simulink model "vertical_smm_with_lqr_3d"  (R2014b)
settings: Solver=FixedStepDiscrete  StartTime=0.0  StopTime=inf  FixedStep=sample_time  RelTol=1e-3
values from neighbouring files (symbols this model uses):
  forward_dx = [-0.304875592207 -0.274388032987 -0.243900473766 -0.213412914545 -0.182925355324 -0.152437796104 -0.121950236883 -0.0914626776622 -0.0609751184415 -0.0304875592207 0 0.0304875592207 ... (714 elements, 21x34)]    [ref_trajs.mat]
  forward_dx_of_dxstar = [-1.3048755994 -1.25487559904 -1.20487559868 -1.15487559832 -1.10487559796 -1.0548755976 -1.00487559724 -0.954875596883 -0.904875596523 -0.854875596164 -0.804875595804 -0.754875595707 ... (29274 elements, 41x21x34)]    [ref_trajs.mat]
  forward_x = [0.0961104217981 0.0864993796183 0.0768883374385 0.0672772952586 0.0576662530788 0.048055210899 0.0384441687192 0.0288331265394 0.0192220843596 0.00961104217981 0 -0.00961104217981 ... (714 elements, 21x34)]    [ref_trajs.mat]
  forward_x_of_dxstar = [0.247353819189 0.239791649319 0.232229479449 0.22466730958 0.21710513971 0.209542969841 0.201980799971 0.194418630102 0.186856460232 0.179294290363 0.171732120493 0.164169950675 ... (29274 elements, 41x21x34)]    [ref_trajs.mat]
  target_dx_range = [-1 -0.95 -0.9 -0.85 -0.8 -0.75 -0.7 -0.65 -0.6 -0.55 -0.5 -0.45 ... (41 elements, 1x41)]    [ref_trajs.mat]
undefined symbols (not defined in the file or in its folder): A_kalman_fourbar_gear, A_kalman_transverse, A_kalman_vertical, A_lpf_dtau, A_lpf_leg_spring, B1_lpf_dtau, B1_lpf_leg_spring, B2_lpf_dtau, B2_lpf_leg_spring, B_dx_versus_x0, B_kalman_fourbar_gear, B_kalman_transverse, B_kalman_vertical, backwards_K_front_of_t_row1, backwards_K_front_of_t_row2, backwards_K_sag_of_t, C_kalman_fourbar_gear, C_kalman_transverse, C_kalman_vertical, com_leg_motor, com_torso, contact_threshold, control_start_time, d_vertical_com, deadbeat_enabled, desired_com_forward_velocity, desired_com_lateral_velocity, desired_initial_leg_roll_left, desired_initial_leg_roll_right, desired_lateral_symmetry_angle, desired_torso_pitch, desired_torso_roll, Discrete, fcut_contact, forward_velocity_target_step, g, HIP_MTR_MAX_CONT_TORQUE, i_leg_motor, i_robot, i_torso, initial_dx_estimate, initial_dy_estimate, initial_dz_estimate, initial_z_estimate, j_motor, j_segments, K_left_lat_flight, K_left_lat_flight_winch, k_LQR_vertical, K_right_lat_flight, K_right_lat_flight_winch, k_sea, k_vertical_winch, kalman_load_to_deflect_transmission, kalman_stance_slip_threshold, kd_motor, kp_motor, l_retract_delta, l_retract_swing_max, l_retract_swing_min ... (+58)
libraries: simulink x8, ctrlSharedLib x7
(part 3 of 4)

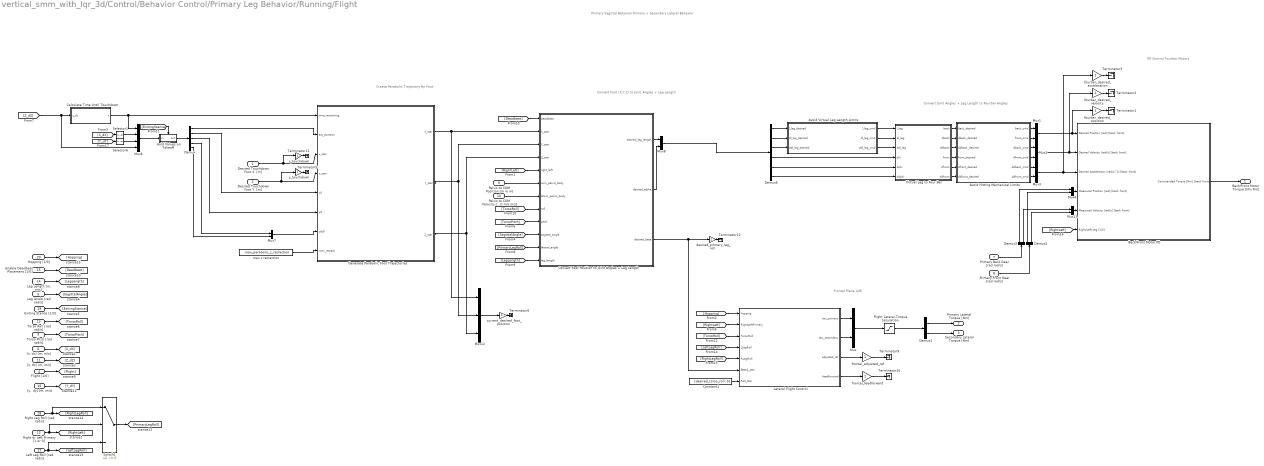
== system vertical_smm_with_lqr_3d/Control/Behavior Control/Primary Leg Behavior/Running/Flight ==
  note: Primary Sagittal Behavior
      | Primary + Secondary Lateral Behavior
  note: Create Parabolic
      | Trajectory for Foot
  note: Convert Foot (X,Y,Z) to
      | Joint Angles + Leg Length
  note: Convert Joint Angles + Leg Length
      | to Fourbar Angles
  note: PD Control Fourbar Motors
  note: Frontal Plane LQR
  Desired Touchdown Foot X  [m] : Inport
  Desired Touchdown Foot Y  [m] : Inport  Port=2
  Torso Pitch [rad rad/s] : Inport  Port=3
  Flight [1/0] : Inport  Port=4
  Leg Angle [rad rad/s] : Inport  Port=5
  "[x, dx] [m, m/s]" : Inport  Port=6
  Primary Back Gear [rad rad/s] : Inport  Port=7
  Primary Front Gear [rad rad/s] : Inport  Port=8
  Pelvis to COM Position [m m m] : Inport  Port=9
  Pelvis to COM Velocity [m/s m/s m/s] : Inport  Port=10
  "[z, dz] [m, m/s]" : Inport  Port=11
  Right or Left Primary [1 or 0] : Inport  Port=12
  Torso Roll [rad rad/s] : Inport  Port=13
  "Leg Length [m, m/s]" : Inport  Port=14
  Enable Deadbeat Placement [1/0] : Inport  Port=15
  "[y,  dy] [m, m/s]" : Inport  Port=16
  "Left Leg Roll [rad, rad/s]" : Inport  Port=17
  "Right Leg Roll [rad, rad/s]" : Inport  Port=18
  Exiting Stance [1/0] : Inport  Port=19
  Hopping [1/0] : Inport  Port=20
  Avoid Hitting Mechanical Limits : MATLAB Function  TreatAsAtomicUnit=on
  Avoid Virtual Leg Length Limits : MATLAB Function  TreatAsAtomicUnit=on
  Back/Front Motor PD : Subsystem
  Calculate Time Until Touchdown : MATLAB Function  TreatAsAtomicUnit=on
  Constant1 : Constant  Value=[desired_torso_roll; 0]
  "Convert Foot Position to Joint Angles + Leg Length " : MATLAB Function  TreatAsAtomicUnit=on
  Demux : Demux  Outputs=5
  Demux1 : Demux  Outputs=2
  Demux2 : Demux  Outputs=2
  Demux3 : Demux  Outputs=2
  Demux6 : Demux  Outputs=6
  Flight Lateral Torque Saturation : Saturate  UpperLimit=HIP_MTR_MAX_CONT_TORQUE  LowerLimit=-HIP_MTR_MAX_CONT_TORQUE
      settings: AttributesFormatString=Top: %<UpperLimit>\nBottom: %<LowerLimit>
  Generate Parabolic Foot Trajectories : MATLAB Function  TreatAsAtomicUnit=on
  Hold Values on Takeoff : Subsystem
  Lateral Flight Control : MATLAB Function  TreatAsAtomicUnit=on
  Mux{,1..4,7..8,11} (8 alike) : Mux  Inputs=2
  Mux12 : Mux  Inputs=3
  Mux6 : Mux
  Selector1 : Selector  InputPortWidth=2  Indices=[1]
  Selector6 : Selector  InputPortWidth=2  Indices=[1]
  Switch1 : Switch  Criteria=u2 ~= 0
  Terminator{1..3,5..6,9..12} (9 alike) : Terminator
  Virtual Leg to Four Bar : MATLAB Function  TreatAsAtomicUnit=on
  current_desired_foot_position : Gain
  desired_primary_leg_roll : Gain
  fourbar_desired_acceleration : Gain
  fourbar_desired_position : Gain
  fourbar_desired_velocity : Gain
  frontal_adjusted_ref : Gain
  frontal_feedforward : Gain
  max z retraction : Constant  Value=max_parabolic_z_retraction
  x_touchdown : Gain
  y_touchdown : Gain
  Back/Front Motor Torque [Nm Nm] : Outport
  Primary Lateral Torque [Nm] : Outport  Port=2
  Secondary Lateral Torque [Nm] : Outport  Port=3
  wires:
  Virtual Leg to Four Bar/1(back) -> Avoid Hitting Mechanical Limits/1(back_desired)
  Virtual Leg to Four Bar/2(dback) -> Avoid Hitting Mechanical Limits/2(dback_desired)
  Virtual Leg to Four Bar/3(ddback) -> Avoid Hitting Mechanical Limits/3(ddback_desired)
  Virtual Leg to Four Bar/4(front) -> Avoid Hitting Mechanical Limits/4(front_desired)
  Virtual Leg to Four Bar/5(dfront) -> Avoid Hitting Mechanical Limits/5(dfront_desired)
  Virtual Leg to Four Bar/6(ddfront) -> Avoid Hitting Mechanical Limits/6(ddfront_desired)
  Mux11/1 -> Back/Front Motor PD/5(Measured Velocity [rad/s] [back front])
  Demux2/2 -> Mux11/2
  Mux4/1 -> Back/Front Motor PD/4(Measured Position [rad] [back front])
  Mux1/1 -> fourbar_desired_position/1, Back/Front Motor PD/1(Desired Position [rad] [back front])
  Demux3/2 -> Mux11/1
  Demux3/1 -> Mux4/1
  Avoid Hitting Mechanical Limits/2(front_cmd) -> Mux1/2
  Avoid Hitting Mechanical Limits/1(back_cmd) -> Mux1/1
  Demux2/1 -> Mux4/2
  Avoid Hitting Mechanical Limits/3(dback_cmd) -> Mux2/1
  Avoid Hitting Mechanical Limits/4(dfront_cmd) -> Mux2/2
  Avoid Hitting Mechanical Limits/5(ddback_cmd) -> Mux3/1
  Avoid Hitting Mechanical Limits/6(ddfront_cmd) -> Mux3/2
  Mux2/1 -> fourbar_desired_velocity/1, Back/Front Motor PD/2(Desired Velocity [rad/s] [back front])
  Mux3/1 -> fourbar_desired_acceleration/1, Back/Front Motor PD/3(Desired Acceleration [rad/s^2] [back front])
  Back/Front Motor PD/1(Commanded Torque [Nm] [back front]) -> Back/Front Motor Torque [Nm Nm]/1
  Primary Back Gear [rad rad/s]/1 -> Demux3/1
  Primary Front Gear [rad rad/s]/1 -> Demux2/1
  [RightLeft] -> Back/Front Motor PD/6(Right/Left Leg [1/0])
  fourbar_desired_position/1 -> Terminator1/1
  fourbar_desired_velocity/1 -> Terminator2/1
  fourbar_desired_acceleration/1 -> Terminator3/1
  Demux/1 -> Generate Parabolic Foot Trajectories/2(est_duration)
  Mux7/1 -> Generate Parabolic Foot Trajectories/7(zdz0)
  max z retraction/1 -> Generate Parabolic Foot Trajectories/8(max_retract)
  Mux6/1 -> Hold Values on Takeoff/1(in)
  Hold Values on Takeoff/1(out) -> Demux/1
  Selector1/1 -> Mux6/2
  [X_dX] -> Selector1/1
  Generate Parabolic Foot Trajectories/1(X_star) -> Mux12/1, "Convert Foot Position to Joint Angles + Leg Length "/2(X_star)
  Generate Parabolic Foot Trajectories/2(Y_star) -> "Convert Foot Position to Joint Angles + Leg Length "/3(Y_star), Mux12/2
  Generate Parabolic Foot Trajectories/3(Z_star) -> "Convert Foot Position to Joint Angles + Leg Length "/4(Z_star), Mux12/3
  [RightLeft] -> "Convert Foot Position to Joint Angles + Leg Length "/5(right_left)
  "Convert Foot Position to Joint Angles + Leg Length "/2(desired_alpha) -> Mux8/2
  "Convert Foot Position to Joint Angles + Leg Length "/1(desired_leg_length) -> Mux8/1
  Demux6/6 -> Virtual Leg to Four Bar/6(ddphi)
  Demux6/5 -> Virtual Leg to Four Bar/5(dphi)
  Demux6/4 -> Virtual Leg to Four Bar/4(phi)
  Mux8/1 -> Demux6/1
  Leg Angle [rad rad/s]/1 -> [SagittalAngle]
  [SagittalAngle] -> "Convert Foot Position to Joint Angles + Leg Length "/10(sagittal_angle)
  Torso Pitch [rad rad/s]/1 -> [TorsoPitch]
  [TorsoPitch] -> "Convert Foot Position to Joint Angles + Leg Length "/9(pitch)
  [PrimaryLegRoll] -> "Convert Foot Position to Joint Angles + Leg Length "/11(lateral_angle)
  [LegLength] -> "Convert Foot Position to Joint Angles + Leg Length "/12(leg_length)
  [TorsoRoll] -> "Convert Foot Position to Joint Angles + Leg Length "/8(roll)
  Pelvis to COM Position [m m m]/1 -> "Convert Foot Position to Joint Angles + Leg Length "/6(com_pelvis_body)
  Pelvis to COM Velocity [m/s m/s m/s]/1 -> "Convert Foot Position to Joint Angles + Leg Length "/7(dcom_pelvis_body)
  Flight [1/0]/1 -> [Flight]
  [ExitingStance] -> Hold Values on Takeoff/Trigger
  "[x, dx] [m, m/s]"/1 -> [X_dX]
  Torso Roll [rad rad/s]/1 -> [TorsoRoll]
  "Leg Length [m, m/s]"/1 -> [LegLength]
  Enable Deadbeat Placement [1/0]/1 -> [Deadbeat]
  "[z, dz] [m, m/s]"/1 -> [Z_dZ]
  Desired Touchdown Foot X  [m]/1 -> x_touchdown/1, Generate Parabolic Foot Trajectories/3(x_star)
  x_touchdown/1 -> Terminator11/1
  y_touchdown/1 -> Terminator5/1
  current_desired_foot_position/1 -> Terminator6/1
  Mux12/1 -> current_desired_foot_position/1
  "[y,  dy] [m, m/s]"/1 -> [Y_dY]
  [Y_dY] -> Selector6/1
  [Z_dZ] -> Mux6/4, Calculate Time Until Touchdown/1(z_dz)
  Selector6/1 -> Mux6/3
  Demux/2 -> Generate Parabolic Foot Trajectories/5(x0)
  Demux/3 -> Generate Parabolic Foot Trajectories/6(y0)
  Demux/4 -> Mux7/1
  Demux/5 -> Mux7/2
  Calculate Time Until Touchdown/1(t) -> Mux6/1, Generate Parabolic Foot Trajectories/1(time_remaining)
  Avoid Virtual Leg Length Limits/1(l_leg_cmd) -> Virtual Leg to Four Bar/1(l_leg)
  Avoid Virtual Leg Length Limits/2(dl_leg_cmd) -> Virtual Leg to Four Bar/2(dl_leg)
  Avoid Virtual Leg Length Limits/3(ddl_leg_cmd) -> Virtual Leg to Four Bar/3(ddl_leg)
  Demux6/1 -> Avoid Virtual Leg Length Limits/1(l_leg_desired)
  Demux6/2 -> Avoid Virtual Leg Length Limits/2(dl_leg_desired)
  Demux6/3 -> Avoid Virtual Leg Length Limits/3(ddl_leg_desired)
  Desired Touchdown Foot Y  [m]/1 -> y_touchdown/1, Generate Parabolic Foot Trajectories/4(y_star)
  [RightLeft] -> Lateral Flight Control/2(RightLeftPrimary)
  [TorsoRoll] -> Lateral Flight Control/3(TorsoRoll)
  Constant1/1 -> Lateral Flight Control/7(Roll_star)
  Lateral Flight Control/3(adjusted_ref) -> frontal_adjusted_ref/1
  Lateral Flight Control/4(feedforward) -> frontal_feedforward/1
  Lateral Flight Control/2(tau_secondary) -> Mux/2
  Lateral Flight Control/1(tau_primary) -> Mux/1
  "Left Leg Roll [rad, rad/s]"/1 -> Switch1/3, [LeftLegRoll]
  [LeftLegRoll] -> Lateral Flight Control/4(LLegRoll)
  [RightLegRoll] -> Lateral Flight Control/5(RLegRoll)
  "Right Leg Roll [rad, rad/s]"/1 -> Switch1/1, [RightLegRoll]
  Right or Left Primary [1 or 0]/1 -> Switch1/2, [RightLeft]
  Switch1/1 -> [PrimaryLegRoll]
  Exiting Stance [1/0]/1 -> [ExitingStance]
  Demux1/1 -> Primary Lateral Torque [Nm]/1
  Demux1/2 -> Secondary Lateral Torque [Nm]/1
  desired_primary_leg_roll/1 -> Terminator12/1
  "Convert Foot Position to Joint Angles + Leg Length "/3(desired_beta) -> Lateral Flight Control/6(Beta1_star), desired_primary_leg_roll/1
  Flight Lateral Torque Saturation/1 -> Demux1/1
  frontal_feedforward/1 -> Terminator10/1
  frontal_adjusted_ref/1 -> Terminator9/1
  [Deadbeat] -> "Convert Foot Position to Joint Angles + Leg Length "/1(deadbeat)
  Mux/1 -> Flight Lateral Torque Saturation/1
  [Hopping] -> Lateral Flight Control/1(hopping)
  Hopping [1/0]/1 -> [Hopping]

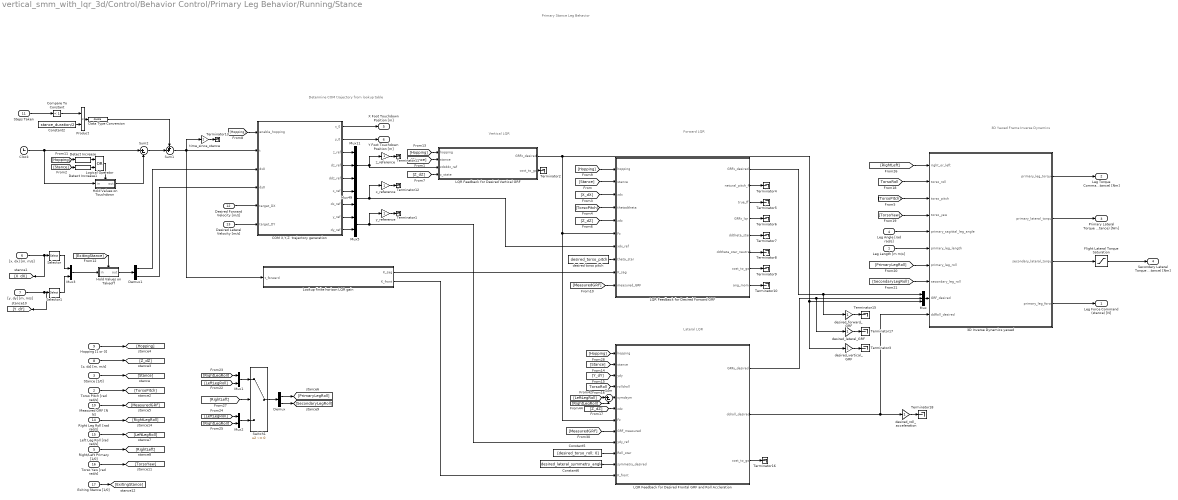
== system vertical_smm_with_lqr_3d/Control/Behavior Control/Primary Leg Behavior/Running/Stance ==
  note: Primary Stance Leg Behavior
  note: Determine COM trajectory
      | from lookup table
  note: Vertical LQR
  note: Forward LQR
  note: 3D Yawed Frame Inverse Dynamics
  note: Lateral LQR
  Leg Length [m m/s] : Inport
  Torso Pitch [rad rad/s] : Inport  Port=2
  Stance [1/0] : Inport  Port=3
  Leg Angle [rad rad/s] : Inport  Port=4
  Right/Left Primary [1/0] : Inport  Port=5
  "[x, dx] [m, m/s]" : Inport  Port=6
  "[y, dy] [m, m/s]" : Inport  Port=7
  "[z, dz] [m, m/s]" : Inport  Port=8
  Hopping [1 or 0] : Inport  Port=9
  Measured GRF [N N] : Inport  Port=10
  Steps Taken : Inport  Port=11
  Desired Forward Velocity [m/s] : Inport  Port=12
  Desired Lateral Velocity [m/s] : Inport  Port=13
  Right Leg Roll [rad rad/s] : Inport  Port=14
  Left Leg Roll [rad rad/s] : Inport  Port=15
  Torso Yaw [rad rad/s] : Inport  Port=16
  Exiting Stance [1/0] : Inport  Port=17
  3D Inverse Dynamics yawed : MATLAB Function  TreatAsAtomicUnit=on
  COM X,Y,Z  trajectory generation : MATLAB Function  TreatAsAtomicUnit=on
  Clock : Clock
  Compare To Constant : simulink/Logic and Bit Operations/Compare To Constant  relop=<  const=1  OutDataTypeStr=uint8
  Constant2 : Constant  Value=stance_duration/2
  Constant5 : Constant  Value=[desired_torso_roll; 0]
  Constant6 : Constant  Value=desired_lateral_symmetry_angle
  Data Type Conversion : DataTypeConversion  OutDataTypeStr=double
  Demux : Demux  Outputs=2
  Demux1 : Demux  Outputs=2
  Detect Increase : simulink/Logic and Bit Operations/Detect Increase  vinit=0.0  InputProcessing=Inherited  OutDataTypeStr=boolean
  Detect Increase1 : simulink/Logic and Bit Operations/Detect Increase  vinit=0.0  InputProcessing=Inherited  OutDataTypeStr=boolean
  Flight Lateral Torque Saturation : Saturate  UpperLimit=HIP_MTR_MAX_CONT_TORQUE  LowerLimit=-HIP_MTR_MAX_CONT_TORQUE
      settings: AttributesFormatString=Top: %<UpperLimit>\nBottom: %<LowerLimit>
  Hold Values on Takeoff : Subsystem
  Hold Values on Touchdown : Subsystem
  LQR Feedback for Desired Forward GRF : MATLAB Function  TreatAsAtomicUnit=on
  LQR Feedback for Desired Frontal GRF and Roll Accleration : MATLAB Function  TreatAsAtomicUnit=on
  LQR Feedback for Desired Vertical GRF : MATLAB Function  TreatAsAtomicUnit=on
  Logical Operator : Logic  Operator=OR  AllPortsSameDT=off  OutDataTypeStr=boolean
  Lookup finite horizon LQR gain : MATLAB Function  TreatAsAtomicUnit=on
  Mux : Mux  Inputs=3
  Mux{1..3,5,49} (5 alike) : Mux  Inputs=2
  Mux11 : Mux  Inputs=3
  Product : Product
  Selector : Selector  InputPortWidth=2  Indices=[2]
  Selector1 : Selector  InputPortWidth=2  Indices=[2]
  Sum : Sum  Inputs=|+-
  Sum1 : Sum  Inputs=++|  OutDataTypeStr=double
  Sum2 : Sum  Inputs=|+-
  Switch1 : Switch  Criteria=u2 ~= 0
  Terminator{1..13,15..18} (17 alike) : Terminator
  desired torso pitch : Constant  Value=desired_torso_pitch
  desired_forward_GRF : Gain
  desired_lateral_GRF : Gain
  desired_roll_acceleration : Gain
  desired_vertical_GRF : Gain
  time_since_stance : Gain
  x_reference : Gain
  y_reference : Gain
  z_reference : Gain
  Leg Force Command (stance) [N] : Outport
  Leg Torque Command (stance) [Nm] : Outport  Port=2
  Primary Lateral Torque Command (stance) [Nm] : Outport  Port=3
  Secondary Lateral Torque Command (stance) [Nm] : Outport  Port=4
  X Foot Touchdown Position [m] : Outport  Port=5
  Y Foot Touchdown Position [m] : Outport  Port=6
  wires:
  3D Inverse Dynamics yawed/1(primary_leg_torque) -> Leg Torque Command (stance) [Nm]/1
  [Z_dZ] -> LQR Feedback for Desired Vertical GRF/4(z_state)
  COM X,Y,Z  trajectory generation/3(z_ref) -> Mux11/1
  [Stance] -> LQR Feedback for Desired Forward GRF/2(stance)
  COM X,Y,Z  trajectory generation/6(x_ref) -> Mux49/1
  COM X,Y,Z  trajectory generation/7(dx_ref) -> Mux49/2
  COM X,Y,Z  trajectory generation/8(y_ref) -> Mux5/1
  COM X,Y,Z  trajectory generation/9(dy_ref) -> Mux5/2
  COM X,Y,Z  trajectory generation/1(x_0) -> X Foot Touchdown Position [m]/1
  COM X,Y,Z  trajectory generation/4(dz_ref) -> Mux11/2
  COM X,Y,Z  trajectory generation/5(ddz_ref) -> Mux11/3
  Mux11/1 -> z_reference/1, LQR Feedback for Desired Vertical GRF/3(zdzddz_ref)
  [X_dX] -> LQR Feedback for Desired Forward GRF/3(xdx)
  [TorsoPitch] -> LQR Feedback for Desired Forward GRF/4(thetadtheta)
  Mux49/1 -> x_reference/1, LQR Feedback for Desired Forward GRF/7(xdx_ref)
  desired torso pitch/1 -> LQR Feedback for Desired Forward GRF/8(theta_star)
  Lookup finite horizon LQR gain/1(K_sag) -> LQR Feedback for Desired Forward GRF/9(K_sag)
  [Z_dZ] -> LQR Feedback for Desired Forward GRF/5(zdz)
  Desired Forward Velocity [m/s]/1 -> COM X,Y,Z  trajectory generation/5(target_DX)
  LQR Feedback for Desired Forward GRF/1(GRFx_desired) -> Mux/1, desired_forward_GRF/1
  Sum1/1 -> Lookup finite horizon LQR gain/1(t_forward), time_since_stance/1, COM X,Y,Z  trajectory generation/2(t)
  LQR Feedback for Desired Vertical GRF/1(GRFz_desired) -> desired_vertical_GRF/1, Mux/3, LQR Feedback for Desired Forward GRF/6(Fz), LQR Feedback for Desired Frontal GRF and Roll Accleration/7(Fz)
  Hold Values on Touchdown/1(out) -> Sum2/2
  Stance [1/0]/1 -> [Stance]
  [Stance] -> LQR Feedback for Desired Vertical GRF/2(stance)
  Logical Operator/1 -> Hold Values on Touchdown/Trigger
  "[x, dx] [m, m/s]"/1 -> [X_dX], Selector/1
  Clock/1 -> Hold Values on Touchdown/1(in), Sum2/1
  Demux1/2 -> COM X,Y,Z  trajectory generation/4(dy0)
  LQR Feedback for Desired Vertical GRF/2(cost_to_go) -> Terminator2/1
  LQR Feedback for Desired Forward GRF/2(netural_pitch_ff) -> Terminator4/1
  LQR Feedback for Desired Forward GRF/3(true_ff) -> Terminator5/1
  LQR Feedback for Desired Forward GRF/4(GRFx_lqr) -> Terminator6/1
  LQR Feedback for Desired Forward GRF/5(ddtheta_star) -> Terminator7/1
  LQR Feedback for Desired Forward GRF/6(ddtheta_star_neutral) -> Terminator8/1
  LQR Feedback for Desired Forward GRF/7(cost_to_go) -> Terminator9/1
  LQR Feedback for Desired Forward GRF/8(ang_mom) -> Terminator10/1
  Torso Pitch [rad rad/s]/1 -> [TorsoPitch]
  [RightLeft] -> 3D Inverse Dynamics yawed/1(right_or_left)
  "[z, dz] [m, m/s]"/1 -> [Z_dZ]
  Hopping [1 or 0]/1 -> [Hopping]
  [Hopping] -> COM X,Y,Z  trajectory generation/1(enable_hopping)
  z_reference/1 -> Terminator11/1
  x_reference/1 -> Terminator12/1
  [Hopping] -> LQR Feedback for Desired Forward GRF/1(hopping)
  Measured GRF [N N]/1 -> [MeasuredGRF]
  [MeasuredGRF] -> LQR Feedback for Desired Forward GRF/10(measured_GRF)
  Steps Taken/1 -> Compare To Constant/1
  Product/1 -> Data Type Conversion/1
  Constant2/1 -> Product/2
  Detect Increase/1 -> Logical Operator/1
  Detect Increase1/1 -> Logical Operator/2
  Compare To Constant/1 -> Product/1
  Sum2/1 -> Sum1/2
  Data Type Conversion/1 -> Sum1/1
  time_since_stance/1 -> Terminator13/1
  [Hopping] -> Detect Increase/1
  [Stance] -> Detect Increase1/1
  Demux1/1 -> COM X,Y,Z  trajectory generation/3(dx0)
  Selector/1 -> Mux3/1
  [Hopping] -> LQR Feedback for Desired Vertical GRF/1(hopping)
  Constant6/1 -> LQR Feedback for Desired Frontal GRF and Roll Accleration/11(symmetry_desired)
  Constant5/1 -> LQR Feedback for Desired Frontal GRF and Roll Accleration/10(Roll_star)
  Lookup finite horizon LQR gain/2(K_front) -> LQR Feedback for Desired Frontal GRF and Roll Accleration/12(K_front)
  LQR Feedback for Desired Frontal GRF and Roll Accleration/3(cost_to_go) -> Terminator16/1
  LQR Feedback for Desired Frontal GRF and Roll Accleration/2(ddroll_desired) -> 3D Inverse Dynamics yawed/10(ddRoll_desired), desired_roll_acceleration/1
  LQR Feedback for Desired Frontal GRF and Roll Accleration/1(GRFy_desired) -> Mux/2, desired_lateral_GRF/1
  [Stance] -> LQR Feedback for Desired Frontal GRF and Roll Accleration/2(stance)
  [Y_dY] -> LQR Feedback for Desired Frontal GRF and Roll Accleration/3(ydy)
  [TorsoRoll] -> LQR Feedback for Desired Frontal GRF and Roll Accleration/4(rolldroll)
  [Z_dZ] -> LQR Feedback for Desired Frontal GRF and Roll Accleration/6(zdz)
  [RightLegRoll] -> Sum/2
  [LeftLegRoll] -> Sum/1
  Sum/1 -> LQR Feedback for Desired Frontal GRF and Roll Accleration/5(symdsym)
  COM X,Y,Z  trajectory generation/2(y_0) -> Y Foot Touchdown Position [m]/1
  Mux5/1 -> y_reference/1, LQR Feedback for Desired Frontal GRF and Roll Accleration/9(ydy_ref)
  y_reference/1 -> Terminator1/1
  Mux/1 -> 3D Inverse Dynamics yawed/9(GRF_desired)
  desired_forward_GRF/1 -> Terminator15/1
  desired_vertical_GRF/1 -> Terminator3/1
  desired_lateral_GRF/1 -> Terminator17/1
  desired_roll_acceleration/1 -> Terminator18/1
  [TorsoPitch] -> 3D Inverse Dynamics yawed/3(torso_pitch)
  [TorsoRoll] -> 3D Inverse Dynamics yawed/2(torso_roll)
  [TorsoYaw] -> 3D Inverse Dynamics yawed/4(torso_yaw)
  Leg Length [m m/s]/1 -> 3D Inverse Dynamics yawed/6(primary_leg_length)
  Leg Angle [rad rad/s]/1 -> 3D Inverse Dynamics yawed/5(primary_sagittal_leg_angle)
  [SecondaryLegRoll] -> 3D Inverse Dynamics yawed/8(secondary_leg_roll)
  [PrimaryLegRoll] -> 3D Inverse Dynamics yawed/7(primary_leg_roll)
  Left Leg Roll [rad rad/s]/1 -> [LeftLegRoll]
  Right/Left Primary [1/0]/1 -> [RightLeft]
  Switch1/1 -> Demux/1
  Demux/2 -> [SecondaryLegRoll]
  Demux/1 -> [PrimaryLegRoll]
  Mux1/1 -> Switch1/1
  Mux2/1 -> Switch1/3
  Right Leg Roll [rad rad/s]/1 -> [RightLegRoll]
  [RightLegRoll] -> Mux1/1
  [LeftLegRoll] -> Mux1/2
  [LeftLegRoll] -> Mux2/1
  [RightLegRoll] -> Mux2/2
  [RightLeft] -> Switch1/2
  "[y, dy] [m, m/s]"/1 -> [Y_dY], Selector1/1
  Mux3/1 -> Hold Values on Takeoff/1(in)
  Hold Values on Takeoff/1(out) -> Demux1/1
  Selector1/1 -> Mux3/2
  Desired Lateral Velocity [m/s]/1 -> COM X,Y,Z  trajectory generation/6(target_DY)
  Torso Yaw [rad rad/s]/1 -> [TorsoYaw]
  Exiting Stance [1/0]/1 -> [ExitingStance]
  [ExitingStance] -> Hold Values on Takeoff/Trigger
  3D Inverse Dynamics yawed/3(secondary_lateral_torque) -> Flight Lateral Torque Saturation/1
  3D Inverse Dynamics yawed/4(primary_leg_force) -> Leg Force Command (stance) [N]/1
  3D Inverse Dynamics yawed/2(primary_lateral_torque) -> Primary Lateral Torque Command (stance) [Nm]/1
  [Hopping] -> LQR Feedback for Desired Frontal GRF and Roll Accleration/1(hopping)
  [MeasuredGRF] -> LQR Feedback for Desired Frontal GRF and Roll Accleration/8(GRF_measured)
  Flight Lateral Torque Saturation/1 -> Secondary Lateral Torque Command (stance) [Nm]/1

== system vertical_smm_with_lqr_3d/Control/Behavior Control/Secondary Leg Behavior/Back//Front Motor PD/Friction Compensation ==
  Right/Left [1/0] : Inport
  Commanded Velocity [rad/s] [back front] : Inport  Port=2
  Product : Product
  Sign : Signum
  Sum1 : Sum
  Switch : Switch  Criteria=u2 ~= 0
  Switch1 : Switch  Criteria=u2 ~= 0
  coulomb_friction_left : Constant  Value=sea_coulomb_friction(3:4)
  coulomb_friction_right : Constant  Value=sea_coulomb_friction(1:2)
  offset_friction_left : Constant  Value=sea_offset_friction(3:4)
  offset_friction_right : Constant  Value=sea_offset_friction(1:2)
  Friction Compensation [Nm] : Outport
  wires:
  Commanded Velocity [rad/s] [back front]/1 -> Sign/1
  Switch/1 -> Sum1/2
  Sum1/1 -> Friction Compensation [Nm]/1
  Product/1 -> Sum1/1
  Right/Left [1/0]/1 -> Switch1/2, Switch/2
  offset_friction_right/1 -> Switch/1
  offset_friction_left/1 -> Switch/3
  coulomb_friction_right/1 -> Switch1/1
  coulomb_friction_left/1 -> Switch1/3
  Switch1/1 -> Product/2
  Sign/1 -> Product/1

== system vertical_smm_with_lqr_3d/Control/Behavior Control/Primary Leg Behavior/Running/Circular Buffer/Enabled on Touchdown ==
  In : Inport
  Enable : EnablePort
  Out : Outport
  wires:
  In/1 -> Out/1

== system vertical_smm_with_lqr_3d/Control/Behavior Control/Primary Leg Behavior/Running/Flight/Back//Front Motor PD ==
  Desired Position [rad] [back front] : Inport
  Desired Velocity [rad/s] [back front] : Inport  Port=2
  Desired Acceleration [rad/s^2] [back front] : Inport  Port=3
  Measured Position [rad] [back front] : Inport  Port=4
  Measured Velocity [rad/s] [back front] : Inport  Port=5
  Right/Left Leg [1/0] : Inport  Port=6
  Friction Compensation : Subsystem
  Product : Product
  Sum1 : Sum  Inputs=|++
  Sum2 : Sum  Inputs=|++
  Sum7 : Sum  Inputs=|+-
  Sum8 : Sum  Inputs=|+-
  Sum9 : Sum
  kd : Gain  Gain=kd_motor
  kp : Gain  Gain=kp_motor
  reflected inertia : Constant  Value=j_motor
  Commanded Torque [Nm] [back front] : Outport
  wires:
  kp/1 -> Sum9/1
  Sum7/1 -> kp/1
  Measured Position [rad] [back front]/1 -> Sum7/2
  Sum9/1 -> Sum1/1
  Sum8/1 -> kd/1
  Desired Position [rad] [back front]/1 -> Sum7/1
  kd/1 -> Sum9/2
  Measured Velocity [rad/s] [back front]/1 -> Sum8/2
  Sum1/1 -> Sum2/1
  Desired Acceleration [rad/s^2] [back front]/1 -> Product/1
  Product/1 -> Sum1/2
  Right/Left Leg [1/0]/1 -> Friction Compensation/1(Right/Left [1/0])
  Sum2/1 -> Commanded Torque [Nm] [back front]/1
  Desired Velocity [rad/s] [back front]/1 -> Friction Compensation/2(Commanded Velocity [rad/s] [back front]), Sum8/1
  reflected inertia/1 -> Product/2
  Friction Compensation/1(Friction Compensation [Nm]) -> Sum2/2

== system vertical_smm_with_lqr_3d/Control/Behavior Control/Primary Leg Behavior/Running/Flight/Hold Values on Takeoff ==
  in : Inport
  Trigger : TriggerPort  ShowOutputPort=on  PortDimensions=1
  Subsystem : Subsystem
  out : Outport
  wires:
  Trigger/1 -> Subsystem/Enable
  Subsystem/1(out) -> out/1
  in/1 -> Subsystem/1(in)

== system vertical_smm_with_lqr_3d/Control/Behavior Control/Primary Leg Behavior/Running/Stance/Hold Values on Takeoff ==
  in : Inport
  Trigger : TriggerPort  ShowOutputPort=on  PortDimensions=1
  Subsystem : Subsystem
  out : Outport
  wires:
  Trigger/1 -> Subsystem/Enable
  Subsystem/1(out) -> out/1
  in/1 -> Subsystem/1(in)

== system vertical_smm_with_lqr_3d/Control/Behavior Control/Primary Leg Behavior/Running/Stance/Hold Values on Touchdown ==
  in : Inport
  Trigger : TriggerPort  ShowOutputPort=on  PortDimensions=1
  Subsystem : Subsystem
  out : Outport
  wires:
  in/1 -> Subsystem/1(in)
  Subsystem/1(out) -> out/1
  Trigger/1 -> Subsystem/Enable

== system vertical_smm_with_lqr_3d/Control/Behavior Control/Primary Leg Behavior/Running/Flight/Back//Front Motor PD/Friction Compensation ==
  Right/Left [1/0] : Inport
  Commanded Velocity [rad/s] [back front] : Inport  Port=2
  Product : Product
  Sign : Signum
  Sum1 : Sum
  Switch : Switch  Criteria=u2 ~= 0
  Switch1 : Switch  Criteria=u2 ~= 0
  coulomb_friction_left : Constant  Value=sea_coulomb_friction(3:4)
  coulomb_friction_right : Constant  Value=sea_coulomb_friction(1:2)
  offset_friction_left : Constant  Value=sea_offset_friction(3:4)
  offset_friction_right : Constant  Value=sea_offset_friction(1:2)
  Friction Compensation [Nm] : Outport
  wires:
  Commanded Velocity [rad/s] [back front]/1 -> Sign/1
  Switch/1 -> Sum1/2
  Sum1/1 -> Friction Compensation [Nm]/1
  Product/1 -> Sum1/1
  Right/Left [1/0]/1 -> Switch1/2, Switch/2
  offset_friction_right/1 -> Switch/1
  offset_friction_left/1 -> Switch/3
  coulomb_friction_right/1 -> Switch1/1
  coulomb_friction_left/1 -> Switch1/3
  Switch1/1 -> Product/2
  Sign/1 -> Product/1

== system vertical_smm_with_lqr_3d/Control/Behavior Control/Primary Leg Behavior/Running/Flight/Hold Values on Takeoff/Subsystem ==
  in : Inport
  Enable : EnablePort
  out : Outport
  wires:
  in/1 -> out/1

== system vertical_smm_with_lqr_3d/Control/Behavior Control/Primary Leg Behavior/Running/Stance/Hold Values on Takeoff/Subsystem ==
  in : Inport
  Enable : EnablePort
  out : Outport
  wires:
  in/1 -> out/1

== system vertical_smm_with_lqr_3d/Control/Behavior Control/Primary Leg Behavior/Running/Stance/Hold Values on Touchdown/Subsystem ==
  in : Inport
  Enable : EnablePort
  out : Outport
  wires:
  in/1 -> out/1

== stateflow chart vertical_smm_with_lqr_3d/Control/Behavior Control/Primary Leg Behavior/State Machine ==
  state TouchDown
  state LockedContact
  state Unloading
  state Takeoff
  state Flight
  (junction 91) -> TouchDown
  TouchDown -> (junction 130) [order 2] : [vertical_grf < contact_threshold]
  (junction 93) -> (junction 91)
  (junction 130) -> (junction 128)
  TouchDown -> LockedContact [order 1] : [vertical_grf > loaded_threshold]
  (junction 115) -> LockedContact
  (junction 118) -> (junction 115)
  LockedContact -> Unloading : [leg_velocity >= 0 && previous_leg_velocity < 0]
  Unloading -> LockedContact [order 2] : [vertical_grf > loaded_threshold && leg_velocity < 0]
  (junction 122) -> (junction 118)
  Unloading -> Takeoff [order 1] : [vertical_grf < contact_threshold || leg_length > max_leg_length]
  Takeoff -> Flight : after(t_flight,sec)
  (default) -> Flight
  Flight -> (junction 93) : [vertical_grf > contact_threshold]
  (junction 128) -> Flight
  data: leg_length input; leg_velocity input; previous_leg_velocity input; vertical_grf input; t_flight parameter; max_leg_length parameter; contact_threshold parameter; loaded_threshold parameter; TouchDown output boolean; LockedContact output boolean; Unloading output boolean; Takeoff output boolean; Flight output boolean

== matlab function vertical_smm_with_lqr_3d/Control/Behavior Control/Primary Leg Behavior/Running/Stance/LQR Feedback for Desired Forward GRF ==
  data: hopping input; stance input; GRFx_desired output; netural_pitch_ff output; true_ff output; GRFx_lqr output; ddtheta_star output; ddtheta_star_neutral output; xdx input; thetadtheta input; zdz input; Fz input; xdx_ref input size=2; theta_star input; K_sag input; measured_GRF input; i_robot parameter; P_LQR_sagittal parameter; cost_to_go output double size=1; ang_mom output
%% LQR for x state

% stance: 1 if in stance, 0 otherwise
% xdx: [ x from stance leg to COM, dx of COM]
% thetadtheta: [pitch, dpitch]
% zdz: [z of COM, dz of COM]
% Fz: Desired z GRF
% xdx_ref: [x, dx] current reference point for COM
% theta_star: desired torso pitch
% K_sag: time dependent LQR gain


% sagittal_state: [x, pitch, dx, dptich]
% theta_star: desired torso pitch


function [GRFx_desired, netural_pitch_ff, true_ff, GRFx_lqr, ddtheta_star, ddtheta_star_neutral, cost_to_go, ang_mom]  =  ...
    LQR_Sagittal(hopping, stance, xdx, thetadtheta, zdz, Fz, xdx_ref, theta_star, K_sag, measured_GRF, i_robot,...
    P_LQR_sagittal)

    sagittal_state = [xdx(1); thetadtheta(1); xdx(2); thetadtheta(2)];
    sagittal_reference = [xdx_ref(1), theta_star, xdx_ref(2), 0]';
    
    % make the target pitch depend on current pitch rate s.t system ends at theta_star after flight
%     sagittal_reference = [xdx_ref(1), theta_star - f_duration*thetadtheta(2), xdx_ref(2), 0]';
    sagittal_error = (sagittal_state - sagittal_reference);
    
   
    GRFx_lqr = - K_sag*sagittal_error;
    cost_to_go = sagittal_error'*P_LQR_sagittal*sagittal_error;
    netural_pitch_ff = Fz*xdx(1)/zdz(1);
    true_ff = Fz*xdx_ref(1)/zdz(1);
    
    if stance == 0
      GRFx_lqr = 0;
      cost_to_go = 0;
      netural_pitch_ff = 0;
      true_ff = 0;
    end
    
    GRFx_desired = netural_pitch_ff + GRFx_lqr;
    if ~hopping % different PD law for lowering off the winch
        GRFx_desired = i_robot/zdz(1)*(-150*(theta_star-thetadtheta(1)) + 30*thetadtheta(2)) + netural_pitch_ff;
    end
    GRFx_desired = min(max(GRFx_desired, -abs(measured_GRF(3))/2), abs(measured_GRF(3))/2); % saturate to friction cone (mu = 0.5)
       
    % quantities for logging
    ddtheta_star_neutral = -(GRFx_lqr)*zdz(1)/i_robot;
    ddtheta_star = -(GRFx_desired - netural_pitch_ff)*zdz(1)/i_robot;
    ang_mom = i_robot*thetadtheta(2);
end

== matlab function vertical_smm_with_lqr_3d/Control/Behavior Control/Torque Distribution Right/Motor Torque Saturation Optimization ==
  data: x1s input; t1 output; x2s input; lambda1 parameter; lambda2 parameter; max_torque_sagittal parameter; t2 output
% Optimal leg motor torque distribution
function [t1, t2] = distribute_torque(x1s, x2s, lambda1, lambda2, max_torque_sagittal)

s = max_torque_sagittal;

% possible solutions
x1 = [                                                      x1s;
                                                            0;
                                                            s;
                                                            0;
                                                           -s;
  (lambda2*s + lambda1*x1s - lambda2*x2s)/(lambda1 + lambda2);
  (lambda1*x1s - lambda2*s + lambda2*x2s)/(lambda1 + lambda2);
  (lambda2*s + lambda1*x1s + lambda2*x2s)/(lambda1 + lambda2);
 -(lambda2*s - lambda1*x1s + lambda2*x2s)/(lambda1 + lambda2)];
 
x2 = [                                                      x2s;
                                                            s;
                                                            0;
                                                           -s;
                                                            0;
  (lambda1*s - lambda1*x1s + lambda2*x2s)/(lambda1 + lambda2);
  (lambda1*s + lambda1*x1s + lambda2*x2s)/(lambda1 + lambda2);
  (lambda1*x1s - lambda1*s + lambda2*x2s)/(lambda1 + lambda2);
 -(lambda1*s + lambda1*x1s - lambda2*x2s)/(lambda1 + lambda2)];

% test constraints
c1 = s - x1 - x2 >= 0;
c2 = s + x1 + x2 >= 0;
c3 = s - x1 + x2 >= 0;
c4 = s + x1 - x2 >= 0;
constraints = c1 & c2 & c3 & c4;

% objective function to maximize
f = -lambda1*(x1-x1s).^2-lambda2*(x2-x2s).^2;
satisfied = find(constraints);
[~,I] = max(f(satisfied));

t1 = x1(satisfied(I));
t2 = x2(satisfied(I));

== matlab function vertical_smm_with_lqr_3d/Control/Behavior Control/Primary Leg Behavior/Running/Stance/LQR Feedback for Desired Frontal GRF and Roll Accleration ==
  data: hopping input; stance input; GRFy_desired output; ydy input; rolldroll input; symdsym input; zdz input; Fz input; GRF_measured input; ydy_ref input; ddroll_desired output; cost_to_go output double size=1; Roll_star input; symmetry_desired input; K_front input; P_LQR_frontal parameter; m_torso parameter; m_leg_motor parameter; lateral_offset parameter; com_torso parameter; i_torso parameter; i_leg_motor parameter
function [GRFy_desired, ddroll_desired, cost_to_go]  =  ...
    LQR_Frontal(hopping, stance, ydy, rolldroll, symdsym, zdz, Fz, GRF_measured,...
           ydy_ref, Roll_star, symmetry_desired, K_front, P_LQR_frontal,...
           m_torso, m_leg_motor, lateral_offset, com_torso, i_torso, i_leg_motor)
    
    % Angular momentum about the pelvis in the frontal plane
    d = norm(com_torso(2:3));
    It_f = i_torso(1);
    Im_f = i_leg_motor(1);
    ang_mom = rolldroll(2)*(m_torso*d^2 + It_f + 2*(m_leg_motor*lateral_offset^2+ Im_f)) -symdsym(2)*(m_leg_motor*lateral_offset^2+Im_f);
    
    frontal_state = [ydy(1); rolldroll(1); symdsym(1); ydy(2); rolldroll(2); ang_mom];
    frontal_reference = [ydy_ref(1); Roll_star(1); symmetry_desired; ydy_ref(2); Roll_star(2); 0];
    frontal_error = frontal_state - frontal_reference;
    % feedforward_Fy = Fz*ydy(1)/zdz(1);
    feedforward_Fy = Fz*ydy_ref(1)/zdz(1);
    u = [feedforward_Fy;0]-K_front*frontal_error;
    
    if ~hopping
        frontal_error([1 4]) = 0;
        u = [Fz*ydy(1)/zdz(1); 0]-K_front*frontal_error;
    end
    
    GRFy_desired = u(1);
    ddroll_desired = u(2);
    cost_to_go = frontal_error'*P_LQR_frontal*frontal_error;
    % saturate to friction cone
    if hopping
        GRFy_desired = min(max(GRFy_desired, -abs(GRF_measured(3))/2), abs(GRF_measured(3))/2);
    else
        GRFy_desired = min(max(GRFy_desired, -0.25*abs(GRF_measured(3))), 0.25*abs(GRF_measured(3)));
    end
    if stance == 0
      GRFy_desired = 0;
      ddroll_desired = 0;
      cost_to_go = 0;
    end
end

== matlab function vertical_smm_with_lqr_3d/Control/Behavior Control/Secondary Leg Behavior/Avoid Hitting Mechanical Limits ==
  data: back_cmd output double; front_cmd output double; dback_cmd output double; dfront_cmd output double; ddback_cmd output double; ddfront_cmd output double; back_desired input; dback_desired input; ddback_desired input; front_desired input; dfront_desired input; ddfront_desired input; min_front_bar_angle parameter; max_front_bar_angle parameter; min_back_bar_angle parameter; max_back_bar_angle parameter
%% Avoid joint limits by ensuring we don't command velocities/accelerations that would push us into them when we are close to them.
function [back_cmd, front_cmd, dback_cmd, dfront_cmd, ddback_cmd, ddfront_cmd] ...
    = AvoidFourbarLimits(back_desired,dback_desired, ddback_desired, ...
          front_desired, dfront_desired, ddfront_desired, ...
          min_front_bar_angle, max_front_bar_angle, min_back_bar_angle, max_back_bar_angle)
    [back_cmd, front_cmd, dback_cmd, dfront_cmd, ddback_cmd, ddfront_cmd] = AvoidFourbarLimits(back_desired,dback_desired, ddback_desired, front_desired, dfront_desired, ddfront_desired, min_front_bar_angle, max_front_bar_angle, min_back_bar_angle, max_back_bar_angle);
end

== matlab function vertical_smm_with_lqr_3d/Control/Behavior Control/State Estimation/PositionUsingRobotGeometry ==
  data: right_left input; horizontal_com_position output; roll input; pitch input; yaw input; horizontal_com_velocity output; lateral_com_position output; lateral_com_velocity output; left_leg_sagittal_angle input; left_leg_lateral_angle input; left_leg_length input; right_leg_sagittal_angle input; right_leg_lateral_angle input; right_leg_length input; m_torso parameter; m_leg_motor parameter; m_leg parameter; com_torso parameter; com_leg_motor parameter; lateral_offset parameter; vertical_com_position output; vertical_com_velocity output; com_left_foot output; dcom_left_foot output; com_right_foot output; dcom_right_foot output; com_pelvis output; dcom_pelvis output
% Returns 2D COM relative to primary foot
function [horizontal_com_position, horizontal_com_velocity, ...
          lateral_com_position, lateral_com_velocity, ...
          vertical_com_position, vertical_com_velocity, ...
          com_left_foot, dcom_left_foot, com_right_foot, dcom_right_foot, ....
          com_pelvis, dcom_pelvis] = ...
         ComPositionUsingRobotGeometry(right_left, ...
                                    roll, pitch, yaw, ...
                                    left_leg_sagittal_angle, left_leg_lateral_angle, left_leg_length, ...
                                    right_leg_sagittal_angle, right_leg_lateral_angle, right_leg_length, ...
                                    m_torso, m_leg_motor, m_leg, com_torso, com_leg_motor, lateral_offset)
                    
    q =  [roll(1), pitch(1), yaw(1), left_leg_sagittal_angle(1), left_leg_lateral_angle(1), left_leg_length(1), right_leg_sagittal_angle(1), right_leg_lateral_angle(1), right_leg_length(1)];
    dq = [roll(2), pitch(2), yaw(2), left_leg_sagittal_angle(2), left_leg_lateral_angle(2), left_leg_length(2), right_leg_sagittal_angle(2), right_leg_lateral_angle(2), right_leg_length(2)];
                    
    [ com_pelvis, dcom_pelvis, ...
      com_left_foot, dcom_left_foot, ...
      com_right_foot, dcom_right_foot ] = ...
    ComCalculationFromRobot( q, dq, m_torso, m_leg_motor, m_leg, com_torso, com_leg_motor, lateral_offset );

    if right_left
        com_position = com_right_foot(4:6);
        com_velocity = dcom_right_foot(4:6);
    else
        com_position = com_left_foot(4:6);
        com_velocity = dcom_left_foot(4:6);
    end


    horizontal_com_position = com_position(1);
    horizontal_com_velocity = com_velocity(1);
    lateral_com_position = com_position(2);
    lateral_com_velocity = com_velocity(2);
    vertical_com_position = com_position(3);
    vertical_com_velocity = com_velocity(3);

end

== matlab function vertical_smm_with_lqr_3d/Control/Behavior Control/Torque Distribution Left/Motor Torque Saturation Optimization ==
  data: x1s input; t1 output; x2s input; lambda1 parameter; lambda2 parameter; max_torque_sagittal parameter; t2 output
% Optimal leg motor torque distribution
function [t1, t2] = distribute_torque(x1s, x2s, lambda1, lambda2, max_torque_sagittal)

s = max_torque_sagittal;

% possible solutions
x1 = [                                                      x1s;
                                                            0;
                                                            s;
                                                            0;
                                                           -s;
  (lambda2*s + lambda1*x1s - lambda2*x2s)/(lambda1 + lambda2);
  (lambda1*x1s - lambda2*s + lambda2*x2s)/(lambda1 + lambda2);
  (lambda2*s + lambda1*x1s + lambda2*x2s)/(lambda1 + lambda2);
 -(lambda2*s - lambda1*x1s + lambda2*x2s)/(lambda1 + lambda2)];
 
x2 = [                                                      x2s;
                                                            s;
                                                            0;
                                                           -s;
                                                            0;
  (lambda1*s - lambda1*x1s + lambda2*x2s)/(lambda1 + lambda2);
  (lambda1*s + lambda1*x1s + lambda2*x2s)/(lambda1 + lambda2);
  (lambda1*x1s - lambda1*s + lambda2*x2s)/(lambda1 + lambda2);
 -(lambda1*s + lambda1*x1s - lambda2*x2s)/(lambda1 + lambda2)];

% test constraints
c1 = s - x1 - x2 >= 0;
c2 = s + x1 + x2 >= 0;
c3 = s - x1 + x2 >= 0;
c4 = s + x1 - x2 >= 0;
constraints = c1 & c2 & c3 & c4;

% objective function to maximize
f = -lambda1*(x1-x1s).^2-lambda2*(x2-x2s).^2;
satisfied = find(constraints);
[~,I] = max(f(satisfied));

t1 = x1(satisfied(I));
t2 = x2(satisfied(I));

== matlab function vertical_smm_with_lqr_3d/Control/Behavior Control/State Estimation/Kalman Filtering/eigen values ==
  data: Z input; E output
function E = eigen(Z)
    E = real(eig(Z));
    E = sort(E);
end

== matlab function vertical_smm_with_lqr_3d/Control/Behavior Control/Primary Leg Behavior/Running/Flight/Generate Parabolic Foot Trajectories ==
  data: time_remaining input; est_duration input; x_star input; y_star input; x0 input; y0 input; zdz0 input; max_retract input; z_land parameter; min_f_duration parameter; X_star output size=3; Y_star output size=3; Z_star output size=3
%% Parabolic trajectory generation for x, y, and z
% est_duration: estimated flight time
% time_remaining: time until estimated touchdown
% stance: 1 if in stance, 0 otherwise
% x_star: desired x for foot to COM
% y_star: desired y for foot to COM
% x0: x position at takeoff
% y0: y position at takeoff
% zdz0: [z, dz] at takeoff
% max_retract: how high to lift z for ground clearance
% z_land: nominal z height for landing
% min_f_duration: minimum trajectory time

function [X_star, Y_star, Z_star]  =  ...
          GenerateParabolicFootTrajectory(time_remaining, est_duration,  ...
                               x_star, y_star, x0, y0, zdz0, ...
                               max_retract,  z_land, min_f_duration)
% we are solving for yawed coordinates xyz of com-foot in flight and
% converting them to joint angles

% estimate z ballistically
% z = z_dz_liftoff(1) + z_dz_liftoff(2)*t_flight -g/2*t_flight^2;
% dz = z_dz_liftoff(2) - g*t_flight;
% 
% z = com_xdx_ydy_zdz(5); dz = com_xdx_ydy_zdz(6);
% time_remaining = (-dz-sqrt(max(dz^2 - 4*g/2*(z_land-z), 0) ) )/ (-g); % ballistic estimate of landing


  % plan a traj from init to desired in estimated duration. Use a
  % discontinuous initial condition if estimated duration too short.
  duration = max(est_duration, min_f_duration);
  t_r = max(min(time_remaining, duration),0);
  % sweep a parabola from x0 to x_star with dx_end = 0
  x_star_t = x_star + (x0-x_star)*(t_r/duration)^2;
  dx_star_t = -(x0-x_star)*2*(t_r/duration)/duration;
  ddx_star_t = (x0-x_star)*2/duration^2;
  % same for y
  y_star_t = y_star + (y0-y_star)*(t_r/duration)^2;
  dy_star_t = -(y0-y_star)*2*(t_r/duration)/duration;
  ddy_star_t = (y0-y_star)*2/duration^2;
  
  % split duration into thirds.  First segment: parabola from z0 to
  % max_retract.  Second and third segments, cos to landing.
  z0 = zdz0(1);
  dt3 = duration / 3;
  z_min = z_land - max_retract;
  if t_r > 2*dt3;
    z_star_t = z_min + (z0-z_min)*((t_r-2*dt3)/dt3)^2;
    dz_star_t = -(z0-z_min)*2*(t_r-2*dt3)/dt3/dt3;
    ddz_star_t = (z0-z_min)*2/dt3^2;
  else
    z_star_t = z_land + (z_min-z_land)/2*(1-cos(t_r/(2*dt3)*pi));
    dz_star_t = -(z_min-z_land)/2*sin(t_r/(2*dt3)*pi)*pi/(2*dt3);
    ddz_star_t = (z_min-z_land)/2*cos(t_r/(2*dt3)*pi)*(pi/(2*dt3))^2;
  end
  % track a sinusoidal z of amplitude max_retract, finishing a half-cycle by t_end
  X_star = [x_star_t; dx_star_t; ddx_star_t];
  Y_star = [y_star_t; dy_star_t; ddy_star_t];
  Z_star = [z_star_t; dz_star_t; ddz_star_t];

== matlab function vertical_smm_with_lqr_3d/Control/Behavior Control/Primary Leg Behavior/Running/Stance/LQR Feedback for Desired Vertical GRF ==
  data: hopping input; stance input; zdzddz_ref input size=3; GRFz_desired output; z_state input; k_LQR_vertical parameter; P_LQR_vertical parameter; k_vertical_winch parameter; m_total_real parameter; g parameter; cost_to_go output double size=1
%% LQR for z during stance

% stance: 1 if in stance, 0 otherwise
% z_state: [z, dz] current estimate
% zdzddz_ref: reference trajectory for z position, velocity, and acceleration


% GRFz_desired: desired z GRF
% cost_to_go: remaining LQR cost

function [GRFz_desired, cost_to_go]   =  ...
               LQR_Vertical_Height(hopping, stance, zdzddz_ref, z_state, ...
                                   k_LQR_vertical, P_LQR_vertical, k_vertical_winch, m_total_real, g)

    z_ref = zdzddz_ref(1:2);     
    ddz_ref = zdzddz_ref(3);
    z_error = (z_state - z_ref);
    GRFz_desired = m_total_real*(g+ddz_ref) - k_LQR_vertical*z_error;
    
    if z_ref(2) < 0
      GRFz_desired = max(50, GRFz_desired);
    end
    
    if ~hopping
        GRFz_desired = m_total_real*g - k_vertical_winch*z_error;
        GRFz_desired = max(200, GRFz_desired);
    end
    
    cost_to_go = z_error'*P_LQR_vertical*z_error;
    
    if stance == 0
      GRFz_desired = 0;
      cost_to_go = 0;
    end
end

== matlab function vertical_smm_with_lqr_3d/Control/Behavior Control/Primary Leg Behavior/Running/Circular Buffer/Buffer6 ==
  data: data input; buffer output size=recorded_steps; trigger input; buffer_size input
function buffer  = buffer_data(data, trigger, buffer_size)

    persistent buffer_memory
    coder.varsize('buffer_memory',100);
    if isempty(buffer_memory)
        buffer_memory = [];
    end
    
    if trigger
        buffer_memory = [data; buffer_memory];
        if size(buffer_memory, 1) > buffer_size
            buffer_memory = buffer_memory(1:buffer_size,:);
        end
    end
    
    buffer = buffer_memory;

end
